simulink model "ddc_dev"  (R2016b)
settings: Solver=VariableStepDiscrete  StartTime=0.0  StopTime=10000  RelTol=1e-3  EnableMultiTasking=on
libraries: xbsIndex_r4 x2641, casper_library_misc x6
(part 6 of 25)

== system ddc_dev/dec_fir1 ==
  sync_in : Inport
  real1 : Inport  Port=2
  imag1 : Inport  Port=3
  real2 : Inport  Port=4
  imag2 : Inport  Port=5
  real3 : Inport  Port=6
  imag3 : Inport  Port=7
  real4 : Inport  Port=8
  imag4 : Inport  Port=9
  real5 : Inport  Port=10
  imag5 : Inport  Port=11
  real6 : Inport  Port=12
  imag6 : Inport  Port=13
  real7 : Inport  Port=14
  imag7 : Inport  Port=15
  real8 : Inport  Port=16
  imag8 : Inport  Port=17
  convert1 : xbsIndex_r4/Convert  gui_display_data_type=Fixed-point  arith_type="Signed  (2's comp)"  n_bits=25  bin_pt=20  float_type=Single  exp_bits=8  fraction_bits=24  quantization="Round  (unbiased: +/- Inf)"  overflow=Wrap  en=off  latency=2  pipeline=off  dbl_ovrd=off  block_type=convert
  convert2 : xbsIndex_r4/Convert  gui_display_data_type=Fixed-point  arith_type="Signed  (2's comp)"  n_bits=25  bin_pt=24  float_type=Single  exp_bits=8  fraction_bits=24  quantization="Round  (unbiased: +/- Inf)"  overflow=Wrap  en=off  latency=2  pipeline=off  dbl_ovrd=off  block_type=convert
  delay : xbsIndex_r4/Delay  rst=off  infoeditControl=Selection of Reset will increase slice count due to use of real FFs and instead of SRLs  en=off  latency=8  reg_retiming=off  dbl_ovrd=off  block_type=delay
      settings: infoedit=Hardware notes: A delay line is a chain, each link of which is an SRL16 or SRL32 followed by a flip-flop.
  fir_dbl_col1 : Subsystem  AncestorBlock=casper_library_downconverter/fir_dbl_col  mask(fir_dbl_col){n_inputs=8, coeff=[-0.0011176 -0.00020448    0.000325  0.00054377  0.00054852  0.00043568  0.00028415  0.00017729], add_latency=1, mult_latency=2, coeff_bit_width=25, coeff_bin_pt=24, first_stage_hdl=on, adder_imp=DSP48}
      mask prompts: n_inputs "Inputs"; coeff "Coefficients"; add_latency "Add latency"; mult_latency "Mult Latency"; coeff_bit_width "Coefficient bit width"; coeff_bin_pt "Coefficient binary point"; first_stage_hdl "Implement first stage of adder trees on output as behavioural HDL"; adder_imp "Adder implementation"
      mask init:
      | fir_dbl_col_init(gcb, ...
      |     'n_inputs', n_inputs, ...
      |     'coeff', coeff, ...
      |     'mult_latency', mult_latency, ...
      |     'add_latency', add_latency, ...
      |     'coeff_bit_width', coeff_bit_width, ...
      |     'coeff_bin_pt', coeff_bin_pt,  ...
      |     'first_stage_hdl', first_stage_hdl, ...
      |     'adder_imp', adder_imp);
      mask Help: eval('xlWeb(''http://casper.berkeley.edu/wiki/Fir_dbl_col'')')
      mask TypeOptions adder_imp: Behavioral | Fabric | DSP48
  fir_dbl_col2 : Subsystem  AncestorBlock=casper_library_downconverter/fir_dbl_col  mask(fir_dbl_col){n_inputs=8, coeff=[-0.0082783  -0.0097532   -0.010008  -0.0092495  -0.0077877  -0.0059668  -0.0041018  -0.0024355], add_latency=1, mult_latency=2, coeff_bit_width=25, coeff_bin_pt=24, first_stage_hdl=on, adder_imp=DSP48}
      mask prompts: n_inputs "Inputs"; coeff "Coefficients"; add_latency "Add latency"; mult_latency "Mult Latency"; coeff_bit_width "Coefficient bit width"; coeff_bin_pt "Coefficient binary point"; first_stage_hdl "Implement first stage of adder trees on output as behavioural HDL"; adder_imp "Adder implementation"
      mask init: same as ddc_dev/dec_fir1/fir_dbl_col1
      mask Help: eval('xlWeb(''http://casper.berkeley.edu/wiki/Fir_dbl_col'')')
      mask TypeOptions adder_imp: Behavioral | Fabric | DSP48
  fir_dbl_col3 : Subsystem  AncestorBlock=casper_library_downconverter/fir_dbl_col  mask(fir_dbl_col){n_inputs=8, coeff=[0.010286    0.012906    0.012956    0.010812   0.0071267   0.0026822  -0.0017544  -0.0055495], add_latency=1, mult_latency=2, coeff_bit_width=25, coeff_bin_pt=24, first_stage_hdl=on, adder_imp=DSP48}
      mask prompts: n_inputs "Inputs"; coeff "Coefficients"; add_latency "Add latency"; mult_latency "Mult Latency"; coeff_bit_width "Coefficient bit width"; coeff_bin_pt "Coefficient binary point"; first_stage_hdl "Implement first stage of adder trees on output as behavioural HDL"; adder_imp "Adder implementation"
      mask init: same as ddc_dev/dec_fir1/fir_dbl_col1
      mask Help: eval('xlWeb(''http://casper.berkeley.edu/wiki/Fir_dbl_col'')')
      mask TypeOptions adder_imp: Behavioral | Fabric | DSP48
  fir_dbl_col4 : Subsystem  AncestorBlock=casper_library_downconverter/fir_dbl_col  mask(fir_dbl_col){n_inputs=8, coeff=[-0.016335   -0.024461   -0.026839   -0.024332   -0.018297   -0.010345  -0.0020805    0.005123], add_latency=1, mult_latency=2, coeff_bit_width=25, coeff_bin_pt=24, first_stage_hdl=on, adder_imp=DSP48}
      mask prompts: n_inputs "Inputs"; coeff "Coefficients"; add_latency "Add latency"; mult_latency "Mult Latency"; coeff_bit_width "Coefficient bit width"; coeff_bin_pt "Coefficient binary point"; first_stage_hdl "Implement first stage of adder trees on output as behavioural HDL"; adder_imp "Adder implementation"
      mask init: same as ddc_dev/dec_fir1/fir_dbl_col1
      mask Help: eval('xlWeb(''http://casper.berkeley.edu/wiki/Fir_dbl_col'')')
      mask TypeOptions adder_imp: Behavioral | Fabric | DSP48
  fir_dbl_col5 : Subsystem  AncestorBlock=casper_library_downconverter/fir_dbl_col  mask(fir_dbl_col){n_inputs=8, coeff=[0.13478      0.1265      0.1109     0.08973    0.065332     0.04028    0.017052  -0.0022894], add_latency=1, mult_latency=2, coeff_bit_width=25, coeff_bin_pt=24, first_stage_hdl=on, adder_imp=DSP48}
      mask prompts: n_inputs "Inputs"; coeff "Coefficients"; add_latency "Add latency"; mult_latency "Mult Latency"; coeff_bit_width "Coefficient bit width"; coeff_bin_pt "Coefficient binary point"; first_stage_hdl "Implement first stage of adder trees on output as behavioural HDL"; adder_imp "Adder implementation"
      mask init: same as ddc_dev/dec_fir1/fir_dbl_col1
      mask Help: eval('xlWeb(''http://casper.berkeley.edu/wiki/Fir_dbl_col'')')
      mask TypeOptions adder_imp: Behavioral | Fabric | DSP48
  imag_sum : Subsystem  AncestorBlock=casper_library_misc/adder_tree  mask(adder_tree){n_inputs=5, latency=1, adder_imp=DSP48, first_stage_hdl=off, floating_point=off, float_type=single, frac_width=0, exp_width=0}
      mask prompts: n_inputs "Number of Inputs"; latency "Add Latency"; adder_imp "Adder implementation"; first_stage_hdl "Use behavioural HDL for first stage of adders"; floating_point "floating point"; float_type "float type"; frac_width "fraction length"; exp_width "exponent length"
      mask help:
      | Sums all inputs using a tree of adds and delays.
      |
      | Number of inputs: The number of inputs to the block to be summed
      | Add latency: The number of clock cycles to perform one addition (affects timing)..
      | Adder implementation: choice of fabric or DSP48E core, or behavioral HDL
      | Use behavioural HDL for first stage of adders: Causes the first stage of adders to be absorbed into DSP blocks if multipliers precede them (Virtex 5). Overrides Adder implementation
      mask init:
      | adder_tree_init(gcb, ...
      |     'n_inputs', n_inputs, ...
      |     'latency', latency, ...
      |     'adder_imp', adder_imp, ...
      |     'floating_point', floating_point, ...
      |     'float_type', float_type, ...
      |     'exp_width', exp_width, ...
      |     'frac_width', frac_width, ...     
      |     'first_stage_hdl', first_stage_hdl);
      settings: AttributesFormatString=latency 3
      mask Help: eval('xlWeb(''http://casper.berkeley.edu/wiki/Adder_tree'')')
      mask TypeOptions adder_imp: Behavioral | Fabric | DSP48
      mask Callback floating_point:
      | onoff = get_param(gcb, 'floating_point');
      | if strcmp(onoff,'on')
      |     enable_fixpt = 'off'
      |     set_param_state(gcb, 'float_type', 'on')
      | 
      |     f_type = get_param(gcb, 'float_type')
      |     if strcmp(f_type,'custom')
      |         set_param_state(gcb, 'exp_width', 'on')
      |         set_param_state(gcb, 'frac_width', 'on')
      |     else
      |         set_param_state(gcb, 'exp_width', 'off')
      |         set_param_state(gcb, 'frac_width', 'off')
      |     end
      | 
      | 
      | else
      |     enable_fixpt = 'on'
      |     set_param_state(gcb, 'float_type', 'off')
      |     set_param_state(gcb, 'exp_width', 'off')
      |     set_param_state(gcb, 'frac_width', 'off')
      | end
      mask TypeOptions float_type: single | custom
      mask Callback float_type:
      | f_type = get_param(gcb, 'float_type')
      | if strcmp(f_type,'custom')
      |     set_param_state(gcb, 'exp_width', 'on')
      |     set_param_state(gcb, 'frac_width', 'on')
      | else
      |     set_param_state(gcb, 'exp_width', 'off')
      |     set_param_state(gcb, 'frac_width', 'off')
      | end
  real_sum : Subsystem  AncestorBlock=casper_library_misc/adder_tree  mask(adder_tree){n_inputs=5, latency=1, adder_imp=DSP48, first_stage_hdl=off, floating_point=off, float_type=single, frac_width=0, exp_width=0}
      mask prompts: n_inputs "Number of Inputs"; latency "Add Latency"; adder_imp "Adder implementation"; first_stage_hdl "Use behavioural HDL for first stage of adders"; floating_point "floating point"; float_type "float type"; frac_width "fraction length"; exp_width "exponent length"
      mask help:
      | Sums all inputs using a tree of adds and delays.
      |
      | Number of inputs: The number of inputs to the block to be summed
      | Add latency: The number of clock cycles to perform one addition (affects timing)..
      | Adder implementation: choice of fabric or DSP48E core, or behavioral HDL
      | Use behavioural HDL for first stage of adders: Causes the first stage of adders to be absorbed into DSP blocks if multipliers precede them (Virtex 5). Overrides Adder implementation
      mask init: same as ddc_dev/dec_fir1/imag_sum
      settings: AttributesFormatString=latency 3
      mask Help: eval('xlWeb(''http://casper.berkeley.edu/wiki/Adder_tree'')')
      mask TypeOptions adder_imp: Behavioral | Fabric | DSP48
      mask Callback floating_point:
      | onoff = get_param(gcb, 'floating_point');
      | if strcmp(onoff,'on')
      |     enable_fixpt = 'off'
      |     set_param_state(gcb, 'float_type', 'on')
      | 
      |     f_type = get_param(gcb, 'float_type')
      |     if strcmp(f_type,'custom')
      |         set_param_state(gcb, 'exp_width', 'on')
      |         set_param_state(gcb, 'frac_width', 'on')
      |     else
      |         set_param_state(gcb, 'exp_width', 'off')
      |         set_param_state(gcb, 'frac_width', 'off')
      |     end
      | 
      | 
      | else
      |     enable_fixpt = 'on'
      |     set_param_state(gcb, 'float_type', 'off')
      |     set_param_state(gcb, 'exp_width', 'off')
      |     set_param_state(gcb, 'frac_width', 'off')
      | end
      mask TypeOptions float_type: single | custom
      mask Callback float_type:
      | f_type = get_param(gcb, 'float_type')
      | if strcmp(f_type,'custom')
      |     set_param_state(gcb, 'exp_width', 'on')
      |     set_param_state(gcb, 'frac_width', 'on')
      | else
      |     set_param_state(gcb, 'exp_width', 'off')
      |     set_param_state(gcb, 'frac_width', 'off')
      | end
  ri_to_c : casper_library_misc/ri_to_c
  shift1 : xbsIndex_r4/Shift  shift_dir=Left  shift_bits=1  en=off  latency=1  precision=Full  arith_type="Signed  (2's comp)"  n_bits=16  bin_pt=14  quantization=Truncate  overflow=Wrap  dbl_ovrd=off  block_type=shift
  shift2 : xbsIndex_r4/Shift  shift_dir=Left  shift_bits=1  en=off  latency=1  precision=Full  arith_type="Signed  (2's comp)"  n_bits=16  bin_pt=14  quantization=Truncate  overflow=Wrap  dbl_ovrd=off  block_type=shift
  sync_out : Outport
  dout : Outport  Port=2
  wires:
  fir_dbl_col5/16(imag_out8) -> fir_dbl_col5/32(imag_back8)
  fir_dbl_col5/15(real_out8) -> fir_dbl_col5/31(real_back8)
  fir_dbl_col5/14(imag_out7) -> fir_dbl_col5/30(imag_back7)
  fir_dbl_col5/13(real_out7) -> fir_dbl_col5/29(real_back7)
  fir_dbl_col5/12(imag_out6) -> fir_dbl_col5/28(imag_back6)
  fir_dbl_col5/11(real_out6) -> fir_dbl_col5/27(real_back6)
  fir_dbl_col5/10(imag_out5) -> fir_dbl_col5/26(imag_back5)
  fir_dbl_col5/9(real_out5) -> fir_dbl_col5/25(real_back5)
  fir_dbl_col5/8(imag_out4) -> fir_dbl_col5/24(imag_back4)
  fir_dbl_col5/7(real_out4) -> fir_dbl_col5/23(real_back4)
  fir_dbl_col5/6(imag_out3) -> fir_dbl_col5/22(imag_back3)
  fir_dbl_col5/5(real_out3) -> fir_dbl_col5/21(real_back3)
  fir_dbl_col5/4(imag_out2) -> fir_dbl_col5/20(imag_back2)
  fir_dbl_col5/3(real_out2) -> fir_dbl_col5/19(real_back2)
  fir_dbl_col5/2(imag_out1) -> fir_dbl_col5/18(imag_back1)
  fir_dbl_col5/1(real_out1) -> fir_dbl_col5/17(real_back1)
  fir_dbl_col5/32(imag_back_out8) -> fir_dbl_col4/32(imag_back8)
  fir_dbl_col5/31(real_back_out8) -> fir_dbl_col4/31(real_back8)
  fir_dbl_col5/30(imag_back_out7) -> fir_dbl_col4/30(imag_back7)
  fir_dbl_col5/29(real_back_out7) -> fir_dbl_col4/29(real_back7)
  fir_dbl_col5/28(imag_back_out6) -> fir_dbl_col4/28(imag_back6)
  fir_dbl_col5/27(real_back_out6) -> fir_dbl_col4/27(real_back6)
  fir_dbl_col5/26(imag_back_out5) -> fir_dbl_col4/26(imag_back5)
  fir_dbl_col5/25(real_back_out5) -> fir_dbl_col4/25(real_back5)
  fir_dbl_col5/24(imag_back_out4) -> fir_dbl_col4/24(imag_back4)
  fir_dbl_col5/23(real_back_out4) -> fir_dbl_col4/23(real_back4)
  fir_dbl_col5/22(imag_back_out3) -> fir_dbl_col4/22(imag_back3)
  fir_dbl_col5/21(real_back_out3) -> fir_dbl_col4/21(real_back3)
  fir_dbl_col5/20(imag_back_out2) -> fir_dbl_col4/20(imag_back2)
  fir_dbl_col5/19(real_back_out2) -> fir_dbl_col4/19(real_back2)
  fir_dbl_col5/18(imag_back_out1) -> fir_dbl_col4/18(imag_back1)
  fir_dbl_col5/17(real_back_out1) -> fir_dbl_col4/17(real_back1)
  fir_dbl_col4/32(imag_back_out8) -> fir_dbl_col3/32(imag_back8)
  fir_dbl_col4/31(real_back_out8) -> fir_dbl_col3/31(real_back8)
  fir_dbl_col4/30(imag_back_out7) -> fir_dbl_col3/30(imag_back7)
  fir_dbl_col4/29(real_back_out7) -> fir_dbl_col3/29(real_back7)
  fir_dbl_col4/28(imag_back_out6) -> fir_dbl_col3/28(imag_back6)
  fir_dbl_col4/27(real_back_out6) -> fir_dbl_col3/27(real_back6)
  fir_dbl_col4/26(imag_back_out5) -> fir_dbl_col3/26(imag_back5)
  fir_dbl_col4/25(real_back_out5) -> fir_dbl_col3/25(real_back5)
  fir_dbl_col4/24(imag_back_out4) -> fir_dbl_col3/24(imag_back4)
  fir_dbl_col4/23(real_back_out4) -> fir_dbl_col3/23(real_back4)
  fir_dbl_col4/22(imag_back_out3) -> fir_dbl_col3/22(imag_back3)
  fir_dbl_col4/21(real_back_out3) -> fir_dbl_col3/21(real_back3)
  fir_dbl_col4/20(imag_back_out2) -> fir_dbl_col3/20(imag_back2)
  fir_dbl_col4/19(real_back_out2) -> fir_dbl_col3/19(real_back2)
  fir_dbl_col4/18(imag_back_out1) -> fir_dbl_col3/18(imag_back1)
  fir_dbl_col4/17(real_back_out1) -> fir_dbl_col3/17(real_back1)
  fir_dbl_col3/32(imag_back_out8) -> fir_dbl_col2/32(imag_back8)
  fir_dbl_col3/31(real_back_out8) -> fir_dbl_col2/31(real_back8)
  fir_dbl_col3/30(imag_back_out7) -> fir_dbl_col2/30(imag_back7)
  fir_dbl_col3/29(real_back_out7) -> fir_dbl_col2/29(real_back7)
  fir_dbl_col3/28(imag_back_out6) -> fir_dbl_col2/28(imag_back6)
  fir_dbl_col3/27(real_back_out6) -> fir_dbl_col2/27(real_back6)
  fir_dbl_col3/26(imag_back_out5) -> fir_dbl_col2/26(imag_back5)
  fir_dbl_col3/25(real_back_out5) -> fir_dbl_col2/25(real_back5)
  fir_dbl_col3/24(imag_back_out4) -> fir_dbl_col2/24(imag_back4)
  fir_dbl_col3/23(real_back_out4) -> fir_dbl_col2/23(real_back4)
  fir_dbl_col3/22(imag_back_out3) -> fir_dbl_col2/22(imag_back3)
  fir_dbl_col3/21(real_back_out3) -> fir_dbl_col2/21(real_back3)
  fir_dbl_col3/20(imag_back_out2) -> fir_dbl_col2/20(imag_back2)
  fir_dbl_col3/19(real_back_out2) -> fir_dbl_col2/19(real_back2)
  fir_dbl_col3/18(imag_back_out1) -> fir_dbl_col2/18(imag_back1)
  fir_dbl_col3/17(real_back_out1) -> fir_dbl_col2/17(real_back1)
  fir_dbl_col2/32(imag_back_out8) -> fir_dbl_col1/32(imag_back8)
  fir_dbl_col2/31(real_back_out8) -> fir_dbl_col1/31(real_back8)
  fir_dbl_col2/30(imag_back_out7) -> fir_dbl_col1/30(imag_back7)
  fir_dbl_col2/29(real_back_out7) -> fir_dbl_col1/29(real_back7)
  fir_dbl_col2/28(imag_back_out6) -> fir_dbl_col1/28(imag_back6)
  fir_dbl_col2/27(real_back_out6) -> fir_dbl_col1/27(real_back6)
  fir_dbl_col2/26(imag_back_out5) -> fir_dbl_col1/26(imag_back5)
  fir_dbl_col2/25(real_back_out5) -> fir_dbl_col1/25(real_back5)
  fir_dbl_col2/24(imag_back_out4) -> fir_dbl_col1/24(imag_back4)
  fir_dbl_col2/23(real_back_out4) -> fir_dbl_col1/23(real_back4)
  fir_dbl_col2/22(imag_back_out3) -> fir_dbl_col1/22(imag_back3)
  fir_dbl_col2/21(real_back_out3) -> fir_dbl_col1/21(real_back3)
  fir_dbl_col2/20(imag_back_out2) -> fir_dbl_col1/20(imag_back2)
  fir_dbl_col2/19(real_back_out2) -> fir_dbl_col1/19(real_back2)
  fir_dbl_col2/18(imag_back_out1) -> fir_dbl_col1/18(imag_back1)
  fir_dbl_col2/17(real_back_out1) -> fir_dbl_col1/17(real_back1)
  real_sum/1(sync_out) -> sync_out/1
  delay/1 -> imag_sum/1(sync), real_sum/1(sync)
  sync_in/1 -> delay/1
  ri_to_c/1 -> dout/1
  convert2/1 -> ri_to_c/2
  convert1/1 -> ri_to_c/1
  shift2/1 -> convert2/1
  shift1/1 -> convert1/1
  imag_sum/2(dout) -> shift2/1
  real_sum/2(dout) -> shift1/1
  fir_dbl_col5/34(imag_sum) -> imag_sum/6(din5)
  fir_dbl_col5/33(real_sum) -> real_sum/6(din5)
  fir_dbl_col4/16(imag_out8) -> fir_dbl_col5/16(imag8)
  fir_dbl_col4/15(real_out8) -> fir_dbl_col5/15(real8)
  fir_dbl_col4/14(imag_out7) -> fir_dbl_col5/14(imag7)
  fir_dbl_col4/13(real_out7) -> fir_dbl_col5/13(real7)
  fir_dbl_col4/12(imag_out6) -> fir_dbl_col5/12(imag6)
  fir_dbl_col4/11(real_out6) -> fir_dbl_col5/11(real6)
  fir_dbl_col4/10(imag_out5) -> fir_dbl_col5/10(imag5)
  fir_dbl_col4/9(real_out5) -> fir_dbl_col5/9(real5)
  fir_dbl_col4/8(imag_out4) -> fir_dbl_col5/8(imag4)
  fir_dbl_col4/7(real_out4) -> fir_dbl_col5/7(real4)
  fir_dbl_col4/6(imag_out3) -> fir_dbl_col5/6(imag3)
  fir_dbl_col4/5(real_out3) -> fir_dbl_col5/5(real3)
  fir_dbl_col4/4(imag_out2) -> fir_dbl_col5/4(imag2)
  fir_dbl_col4/3(real_out2) -> fir_dbl_col5/3(real2)
  fir_dbl_col4/2(imag_out1) -> fir_dbl_col5/2(imag1)
  fir_dbl_col4/1(real_out1) -> fir_dbl_col5/1(real1)
  fir_dbl_col4/34(imag_sum) -> imag_sum/5(din4)
  fir_dbl_col4/33(real_sum) -> real_sum/5(din4)
  fir_dbl_col3/16(imag_out8) -> fir_dbl_col4/16(imag8)
  fir_dbl_col3/15(real_out8) -> fir_dbl_col4/15(real8)
  fir_dbl_col3/14(imag_out7) -> fir_dbl_col4/14(imag7)
  fir_dbl_col3/13(real_out7) -> fir_dbl_col4/13(real7)
  fir_dbl_col3/12(imag_out6) -> fir_dbl_col4/12(imag6)
  fir_dbl_col3/11(real_out6) -> fir_dbl_col4/11(real6)
  fir_dbl_col3/10(imag_out5) -> fir_dbl_col4/10(imag5)
  fir_dbl_col3/9(real_out5) -> fir_dbl_col4/9(real5)
  fir_dbl_col3/8(imag_out4) -> fir_dbl_col4/8(imag4)
  fir_dbl_col3/7(real_out4) -> fir_dbl_col4/7(real4)
  fir_dbl_col3/6(imag_out3) -> fir_dbl_col4/6(imag3)
  fir_dbl_col3/5(real_out3) -> fir_dbl_col4/5(real3)
  fir_dbl_col3/4(imag_out2) -> fir_dbl_col4/4(imag2)
  fir_dbl_col3/3(real_out2) -> fir_dbl_col4/3(real2)
  fir_dbl_col3/2(imag_out1) -> fir_dbl_col4/2(imag1)
  fir_dbl_col3/1(real_out1) -> fir_dbl_col4/1(real1)
  fir_dbl_col3/34(imag_sum) -> imag_sum/4(din3)
  fir_dbl_col3/33(real_sum) -> real_sum/4(din3)
  fir_dbl_col2/16(imag_out8) -> fir_dbl_col3/16(imag8)
  fir_dbl_col2/15(real_out8) -> fir_dbl_col3/15(real8)
  fir_dbl_col2/14(imag_out7) -> fir_dbl_col3/14(imag7)
  fir_dbl_col2/13(real_out7) -> fir_dbl_col3/13(real7)
  fir_dbl_col2/12(imag_out6) -> fir_dbl_col3/12(imag6)
  fir_dbl_col2/11(real_out6) -> fir_dbl_col3/11(real6)
  fir_dbl_col2/10(imag_out5) -> fir_dbl_col3/10(imag5)
  fir_dbl_col2/9(real_out5) -> fir_dbl_col3/9(real5)
  fir_dbl_col2/8(imag_out4) -> fir_dbl_col3/8(imag4)
  fir_dbl_col2/7(real_out4) -> fir_dbl_col3/7(real4)
  fir_dbl_col2/6(imag_out3) -> fir_dbl_col3/6(imag3)
  fir_dbl_col2/5(real_out3) -> fir_dbl_col3/5(real3)
  fir_dbl_col2/4(imag_out2) -> fir_dbl_col3/4(imag2)
  fir_dbl_col2/3(real_out2) -> fir_dbl_col3/3(real2)
  fir_dbl_col2/2(imag_out1) -> fir_dbl_col3/2(imag1)
  fir_dbl_col2/1(real_out1) -> fir_dbl_col3/1(real1)
  fir_dbl_col2/34(imag_sum) -> imag_sum/3(din2)
  fir_dbl_col2/33(real_sum) -> real_sum/3(din2)
  fir_dbl_col1/16(imag_out8) -> fir_dbl_col2/16(imag8)
  fir_dbl_col1/15(real_out8) -> fir_dbl_col2/15(real8)
  fir_dbl_col1/14(imag_out7) -> fir_dbl_col2/14(imag7)
  fir_dbl_col1/13(real_out7) -> fir_dbl_col2/13(real7)
  fir_dbl_col1/12(imag_out6) -> fir_dbl_col2/12(imag6)
  fir_dbl_col1/11(real_out6) -> fir_dbl_col2/11(real6)
  fir_dbl_col1/10(imag_out5) -> fir_dbl_col2/10(imag5)
  fir_dbl_col1/9(real_out5) -> fir_dbl_col2/9(real5)
  fir_dbl_col1/8(imag_out4) -> fir_dbl_col2/8(imag4)
  fir_dbl_col1/7(real_out4) -> fir_dbl_col2/7(real4)
  fir_dbl_col1/6(imag_out3) -> fir_dbl_col2/6(imag3)
  fir_dbl_col1/5(real_out3) -> fir_dbl_col2/5(real3)
  fir_dbl_col1/4(imag_out2) -> fir_dbl_col2/4(imag2)
  fir_dbl_col1/3(real_out2) -> fir_dbl_col2/3(real2)
  fir_dbl_col1/2(imag_out1) -> fir_dbl_col2/2(imag1)
  fir_dbl_col1/1(real_out1) -> fir_dbl_col2/1(real1)
  fir_dbl_col1/34(imag_sum) -> imag_sum/2(din1)
  fir_dbl_col1/33(real_sum) -> real_sum/2(din1)
  imag8/1 -> fir_dbl_col1/16(imag8)
  real8/1 -> fir_dbl_col1/15(real8)
  imag7/1 -> fir_dbl_col1/14(imag7)
  real7/1 -> fir_dbl_col1/13(real7)
  imag6/1 -> fir_dbl_col1/12(imag6)
  real6/1 -> fir_dbl_col1/11(real6)
  imag5/1 -> fir_dbl_col1/10(imag5)
  real5/1 -> fir_dbl_col1/9(real5)
  imag4/1 -> fir_dbl_col1/8(imag4)
  real4/1 -> fir_dbl_col1/7(real4)
  imag3/1 -> fir_dbl_col1/6(imag3)
  real3/1 -> fir_dbl_col1/5(real3)
  imag2/1 -> fir_dbl_col1/4(imag2)
  real2/1 -> fir_dbl_col1/3(real2)
  imag1/1 -> fir_dbl_col1/2(imag1)
  real1/1 -> fir_dbl_col1/1(real1)

== system ddc_dev/dec_fir2 ==
  sync_in : Inport
  real1 : Inport  Port=2
  imag1 : Inport  Port=3
  real2 : Inport  Port=4
  imag2 : Inport  Port=5
  real3 : Inport  Port=6
  imag3 : Inport  Port=7
  real4 : Inport  Port=8
  imag4 : Inport  Port=9
  real5 : Inport  Port=10
  imag5 : Inport  Port=11
  real6 : Inport  Port=12
  imag6 : Inport  Port=13
  real7 : Inport  Port=14
  imag7 : Inport  Port=15
  real8 : Inport  Port=16
  imag8 : Inport  Port=17
  convert1 : xbsIndex_r4/Convert  gui_display_data_type=Fixed-point  arith_type="Signed  (2's comp)"  n_bits=25  bin_pt=20  float_type=Single  exp_bits=8  fraction_bits=24  quantization="Round  (unbiased: +/- Inf)"  overflow=Wrap  en=off  latency=2  pipeline=off  dbl_ovrd=off  block_type=convert
  convert2 : xbsIndex_r4/Convert  gui_display_data_type=Fixed-point  arith_type="Signed  (2's comp)"  n_bits=25  bin_pt=24  float_type=Single  exp_bits=8  fraction_bits=24  quantization="Round  (unbiased: +/- Inf)"  overflow=Wrap  en=off  latency=2  pipeline=off  dbl_ovrd=off  block_type=convert
  delay : xbsIndex_r4/Delay  rst=off  infoeditControl=Selection of Reset will increase slice count due to use of real FFs and instead of SRLs  en=off  latency=8  reg_retiming=off  dbl_ovrd=off  block_type=delay
      settings: infoedit=Hardware notes: A delay line is a chain, each link of which is an SRL16 or SRL32 followed by a flip-flop.
  fir_dbl_col1 : Subsystem  AncestorBlock=casper_library_downconverter/fir_dbl_col  mask(fir_dbl_col){n_inputs=8, coeff=[-0.0011176 -0.00020448    0.000325  0.00054377  0.00054852  0.00043568  0.00028415  0.00017729], add_latency=1, mult_latency=2, coeff_bit_width=25, coeff_bin_pt=24, first_stage_hdl=on, adder_imp=DSP48}
      mask prompts: n_inputs "Inputs"; coeff "Coefficients"; add_latency "Add latency"; mult_latency "Mult Latency"; coeff_bit_width "Coefficient bit width"; coeff_bin_pt "Coefficient binary point"; first_stage_hdl "Implement first stage of adder trees on output as behavioural HDL"; adder_imp "Adder implementation"
      mask init: same as ddc_dev/dec_fir1/fir_dbl_col1
      mask Help: eval('xlWeb(''http://casper.berkeley.edu/wiki/Fir_dbl_col'')')
      mask TypeOptions adder_imp: Behavioral | Fabric | DSP48
  fir_dbl_col2 : Subsystem  AncestorBlock=casper_library_downconverter/fir_dbl_col  mask(fir_dbl_col){n_inputs=8, coeff=[-0.0082783  -0.0097532   -0.010008  -0.0092495  -0.0077877  -0.0059668  -0.0041018  -0.0024355], add_latency=1, mult_latency=2, coeff_bit_width=25, coeff_bin_pt=24, first_stage_hdl=on, adder_imp=DSP48}
      mask prompts: n_inputs "Inputs"; coeff "Coefficients"; add_latency "Add latency"; mult_latency "Mult Latency"; coeff_bit_width "Coefficient bit width"; coeff_bin_pt "Coefficient binary point"; first_stage_hdl "Implement first stage of adder trees on output as behavioural HDL"; adder_imp "Adder implementation"
      mask init: same as ddc_dev/dec_fir1/fir_dbl_col1
      mask Help: eval('xlWeb(''http://casper.berkeley.edu/wiki/Fir_dbl_col'')')
      mask TypeOptions adder_imp: Behavioral | Fabric | DSP48
  fir_dbl_col3 : Subsystem  AncestorBlock=casper_library_downconverter/fir_dbl_col  mask(fir_dbl_col){n_inputs=8, coeff=[0.010286    0.012906    0.012956    0.010812   0.0071267   0.0026822  -0.0017544  -0.0055495], add_latency=1, mult_latency=2, coeff_bit_width=25, coeff_bin_pt=24, first_stage_hdl=on, adder_imp=DSP48}
      mask prompts: n_inputs "Inputs"; coeff "Coefficients"; add_latency "Add latency"; mult_latency "Mult Latency"; coeff_bit_width "Coefficient bit width"; coeff_bin_pt "Coefficient binary point"; first_stage_hdl "Implement first stage of adder trees on output as behavioural HDL"; adder_imp "Adder implementation"
      mask init: same as ddc_dev/dec_fir1/fir_dbl_col1
      mask Help: eval('xlWeb(''http://casper.berkeley.edu/wiki/Fir_dbl_col'')')
      mask TypeOptions adder_imp: Behavioral | Fabric | DSP48
  fir_dbl_col4 : Subsystem  AncestorBlock=casper_library_downconverter/fir_dbl_col  mask(fir_dbl_col){n_inputs=8, coeff=[-0.016335   -0.024461   -0.026839   -0.024332   -0.018297   -0.010345  -0.0020805    0.005123], add_latency=1, mult_latency=2, coeff_bit_width=25, coeff_bin_pt=24, first_stage_hdl=on, adder_imp=DSP48}
      mask prompts: n_inputs "Inputs"; coeff "Coefficients"; add_latency "Add latency"; mult_latency "Mult Latency"; coeff_bit_width "Coefficient bit width"; coeff_bin_pt "Coefficient binary point"; first_stage_hdl "Implement first stage of adder trees on output as behavioural HDL"; adder_imp "Adder implementation"
      mask init: same as ddc_dev/dec_fir1/fir_dbl_col1
      mask Help: eval('xlWeb(''http://casper.berkeley.edu/wiki/Fir_dbl_col'')')
      mask TypeOptions adder_imp: Behavioral | Fabric | DSP48
  fir_dbl_col5 : Subsystem  AncestorBlock=casper_library_downconverter/fir_dbl_col  mask(fir_dbl_col){n_inputs=8, coeff=[0.13478      0.1265      0.1109     0.08973    0.065332     0.04028    0.017052  -0.0022894], add_latency=1, mult_latency=2, coeff_bit_width=25, coeff_bin_pt=24, first_stage_hdl=on, adder_imp=DSP48}
      mask prompts: n_inputs "Inputs"; coeff "Coefficients"; add_latency "Add latency"; mult_latency "Mult Latency"; coeff_bit_width "Coefficient bit width"; coeff_bin_pt "Coefficient binary point"; first_stage_hdl "Implement first stage of adder trees on output as behavioural HDL"; adder_imp "Adder implementation"
      mask init: same as ddc_dev/dec_fir1/fir_dbl_col1
      mask Help: eval('xlWeb(''http://casper.berkeley.edu/wiki/Fir_dbl_col'')')
      mask TypeOptions adder_imp: Behavioral | Fabric | DSP48
  imag_sum : Subsystem  AncestorBlock=casper_library_misc/adder_tree  mask(adder_tree){n_inputs=5, latency=1, adder_imp=DSP48, first_stage_hdl=off, floating_point=off, float_type=single, frac_width=0, exp_width=0}
      mask prompts: n_inputs "Number of Inputs"; latency "Add Latency"; adder_imp "Adder implementation"; first_stage_hdl "Use behavioural HDL for first stage of adders"; floating_point "floating point"; float_type "float type"; frac_width "fraction length"; exp_width "exponent length"
      mask help:
      | Sums all inputs using a tree of adds and delays.
      |
      | Number of inputs: The number of inputs to the block to be summed
      | Add latency: The number of clock cycles to perform one addition (affects timing)..
      | Adder implementation: choice of fabric or DSP48E core, or behavioral HDL
      | Use behavioural HDL for first stage of adders: Causes the first stage of adders to be absorbed into DSP blocks if multipliers precede them (Virtex 5). Overrides Adder implementation
      mask init: same as ddc_dev/dec_fir1/imag_sum
      settings: AttributesFormatString=latency 3
      mask Help: eval('xlWeb(''http://casper.berkeley.edu/wiki/Adder_tree'')')
      mask TypeOptions adder_imp: Behavioral | Fabric | DSP48
      mask Callback floating_point:
      | onoff = get_param(gcb, 'floating_point');
      | if strcmp(onoff,'on')
      |     enable_fixpt = 'off'
      |     set_param_state(gcb, 'float_type', 'on')
      | 
      |     f_type = get_param(gcb, 'float_type')
      |     if strcmp(f_type,'custom')
      |         set_param_state(gcb, 'exp_width', 'on')
      |         set_param_state(gcb, 'frac_width', 'on')
      |     else
      |         set_param_state(gcb, 'exp_width', 'off')
      |         set_param_state(gcb, 'frac_width', 'off')
      |     end
      | 
      | 
      | else
      |     enable_fixpt = 'on'
      |     set_param_state(gcb, 'float_type', 'off')
      |     set_param_state(gcb, 'exp_width', 'off')
      |     set_param_state(gcb, 'frac_width', 'off')
      | end
      mask TypeOptions float_type: single | custom
      mask Callback float_type:
      | f_type = get_param(gcb, 'float_type')
      | if strcmp(f_type,'custom')
      |     set_param_state(gcb, 'exp_width', 'on')
      |     set_param_state(gcb, 'frac_width', 'on')
      | else
      |     set_param_state(gcb, 'exp_width', 'off')
      |     set_param_state(gcb, 'frac_width', 'off')
      | end
  real_sum : Subsystem  AncestorBlock=casper_library_misc/adder_tree  mask(adder_tree){n_inputs=5, latency=1, adder_imp=DSP48, first_stage_hdl=off, floating_point=off, float_type=single, frac_width=0, exp_width=0}
      mask prompts: n_inputs "Number of Inputs"; latency "Add Latency"; adder_imp "Adder implementation"; first_stage_hdl "Use behavioural HDL for first stage of adders"; floating_point "floating point"; float_type "float type"; frac_width "fraction length"; exp_width "exponent length"
      mask help:
      | Sums all inputs using a tree of adds and delays.
      |
      | Number of inputs: The number of inputs to the block to be summed
      | Add latency: The number of clock cycles to perform one addition (affects timing)..
      | Adder implementation: choice of fabric or DSP48E core, or behavioral HDL
      | Use behavioural HDL for first stage of adders: Causes the first stage of adders to be absorbed into DSP blocks if multipliers precede them (Virtex 5). Overrides Adder implementation
      mask init: same as ddc_dev/dec_fir1/imag_sum
      settings: AttributesFormatString=latency 3
      mask Help: eval('xlWeb(''http://casper.berkeley.edu/wiki/Adder_tree'')')
      mask TypeOptions adder_imp: Behavioral | Fabric | DSP48
      mask Callback floating_point:
      | onoff = get_param(gcb, 'floating_point');
      | if strcmp(onoff,'on')
      |     enable_fixpt = 'off'
      |     set_param_state(gcb, 'float_type', 'on')
      | 
      |     f_type = get_param(gcb, 'float_type')
      |     if strcmp(f_type,'custom')
      |         set_param_state(gcb, 'exp_width', 'on')
      |         set_param_state(gcb, 'frac_width', 'on')
      |     else
      |         set_param_state(gcb, 'exp_width', 'off')
      |         set_param_state(gcb, 'frac_width', 'off')
      |     end
      | 
      | 
      | else
      |     enable_fixpt = 'on'
      |     set_param_state(gcb, 'float_type', 'off')
      |     set_param_state(gcb, 'exp_width', 'off')
      |     set_param_state(gcb, 'frac_width', 'off')
      | end
      mask TypeOptions float_type: single | custom
      mask Callback float_type:
      | f_type = get_param(gcb, 'float_type')
      | if strcmp(f_type,'custom')
      |     set_param_state(gcb, 'exp_width', 'on')
      |     set_param_state(gcb, 'frac_width', 'on')
      | else
      |     set_param_state(gcb, 'exp_width', 'off')
      |     set_param_state(gcb, 'frac_width', 'off')
      | end
  ri_to_c : casper_library_misc/ri_to_c
  shift1 : xbsIndex_r4/Shift  shift_dir=Left  shift_bits=1  en=off  latency=1  precision=Full  arith_type="Signed  (2's comp)"  n_bits=16  bin_pt=14  quantization=Truncate  overflow=Wrap  dbl_ovrd=off  block_type=shift
  shift2 : xbsIndex_r4/Shift  shift_dir=Left  shift_bits=1  en=off  latency=1  precision=Full  arith_type="Signed  (2's comp)"  n_bits=16  bin_pt=14  quantization=Truncate  overflow=Wrap  dbl_ovrd=off  block_type=shift
  sync_out : Outport
  dout : Outport  Port=2
  wires:
  real1/1 -> fir_dbl_col1/1(real1)
  imag1/1 -> fir_dbl_col1/2(imag1)
  real2/1 -> fir_dbl_col1/3(real2)
  imag2/1 -> fir_dbl_col1/4(imag2)
  real3/1 -> fir_dbl_col1/5(real3)
  imag3/1 -> fir_dbl_col1/6(imag3)
  real4/1 -> fir_dbl_col1/7(real4)
  imag4/1 -> fir_dbl_col1/8(imag4)
  real5/1 -> fir_dbl_col1/9(real5)
  imag5/1 -> fir_dbl_col1/10(imag5)
  real6/1 -> fir_dbl_col1/11(real6)
  imag6/1 -> fir_dbl_col1/12(imag6)
  real7/1 -> fir_dbl_col1/13(real7)
  imag7/1 -> fir_dbl_col1/14(imag7)
  real8/1 -> fir_dbl_col1/15(real8)
  imag8/1 -> fir_dbl_col1/16(imag8)
  fir_dbl_col1/33(real_sum) -> real_sum/2(din1)
  fir_dbl_col1/34(imag_sum) -> imag_sum/2(din1)
  fir_dbl_col1/1(real_out1) -> fir_dbl_col2/1(real1)
  fir_dbl_col1/2(imag_out1) -> fir_dbl_col2/2(imag1)
  fir_dbl_col1/3(real_out2) -> fir_dbl_col2/3(real2)
  fir_dbl_col1/4(imag_out2) -> fir_dbl_col2/4(imag2)
  fir_dbl_col1/5(real_out3) -> fir_dbl_col2/5(real3)
  fir_dbl_col1/6(imag_out3) -> fir_dbl_col2/6(imag3)
  fir_dbl_col1/7(real_out4) -> fir_dbl_col2/7(real4)
  fir_dbl_col1/8(imag_out4) -> fir_dbl_col2/8(imag4)
  fir_dbl_col1/9(real_out5) -> fir_dbl_col2/9(real5)
  fir_dbl_col1/10(imag_out5) -> fir_dbl_col2/10(imag5)
  fir_dbl_col1/11(real_out6) -> fir_dbl_col2/11(real6)
  fir_dbl_col1/12(imag_out6) -> fir_dbl_col2/12(imag6)
  fir_dbl_col1/13(real_out7) -> fir_dbl_col2/13(real7)
  fir_dbl_col1/14(imag_out7) -> fir_dbl_col2/14(imag7)
  fir_dbl_col1/15(real_out8) -> fir_dbl_col2/15(real8)
  fir_dbl_col1/16(imag_out8) -> fir_dbl_col2/16(imag8)
  fir_dbl_col2/33(real_sum) -> real_sum/3(din2)
  fir_dbl_col2/34(imag_sum) -> imag_sum/3(din2)
  fir_dbl_col2/1(real_out1) -> fir_dbl_col3/1(real1)
  fir_dbl_col2/2(imag_out1) -> fir_dbl_col3/2(imag1)
  fir_dbl_col2/3(real_out2) -> fir_dbl_col3/3(real2)
  fir_dbl_col2/4(imag_out2) -> fir_dbl_col3/4(imag2)
  fir_dbl_col2/5(real_out3) -> fir_dbl_col3/5(real3)
  fir_dbl_col2/6(imag_out3) -> fir_dbl_col3/6(imag3)
  fir_dbl_col2/7(real_out4) -> fir_dbl_col3/7(real4)
  fir_dbl_col2/8(imag_out4) -> fir_dbl_col3/8(imag4)
  fir_dbl_col2/9(real_out5) -> fir_dbl_col3/9(real5)
  fir_dbl_col2/10(imag_out5) -> fir_dbl_col3/10(imag5)
  fir_dbl_col2/11(real_out6) -> fir_dbl_col3/11(real6)
  fir_dbl_col2/12(imag_out6) -> fir_dbl_col3/12(imag6)
  fir_dbl_col2/13(real_out7) -> fir_dbl_col3/13(real7)
  fir_dbl_col2/14(imag_out7) -> fir_dbl_col3/14(imag7)
  fir_dbl_col2/15(real_out8) -> fir_dbl_col3/15(real8)
  fir_dbl_col2/16(imag_out8) -> fir_dbl_col3/16(imag8)
  fir_dbl_col3/33(real_sum) -> real_sum/4(din3)
  fir_dbl_col3/34(imag_sum) -> imag_sum/4(din3)
  fir_dbl_col3/1(real_out1) -> fir_dbl_col4/1(real1)
  fir_dbl_col3/2(imag_out1) -> fir_dbl_col4/2(imag1)
  fir_dbl_col3/3(real_out2) -> fir_dbl_col4/3(real2)
  fir_dbl_col3/4(imag_out2) -> fir_dbl_col4/4(imag2)
  fir_dbl_col3/5(real_out3) -> fir_dbl_col4/5(real3)
  fir_dbl_col3/6(imag_out3) -> fir_dbl_col4/6(imag3)
  fir_dbl_col3/7(real_out4) -> fir_dbl_col4/7(real4)
  fir_dbl_col3/8(imag_out4) -> fir_dbl_col4/8(imag4)
  fir_dbl_col3/9(real_out5) -> fir_dbl_col4/9(real5)
  fir_dbl_col3/10(imag_out5) -> fir_dbl_col4/10(imag5)
  fir_dbl_col3/11(real_out6) -> fir_dbl_col4/11(real6)
  fir_dbl_col3/12(imag_out6) -> fir_dbl_col4/12(imag6)
  fir_dbl_col3/13(real_out7) -> fir_dbl_col4/13(real7)
  fir_dbl_col3/14(imag_out7) -> fir_dbl_col4/14(imag7)
  fir_dbl_col3/15(real_out8) -> fir_dbl_col4/15(real8)
  fir_dbl_col3/16(imag_out8) -> fir_dbl_col4/16(imag8)
  fir_dbl_col4/33(real_sum) -> real_sum/5(din4)
  fir_dbl_col4/34(imag_sum) -> imag_sum/5(din4)
  fir_dbl_col4/1(real_out1) -> fir_dbl_col5/1(real1)
  fir_dbl_col4/2(imag_out1) -> fir_dbl_col5/2(imag1)
  fir_dbl_col4/3(real_out2) -> fir_dbl_col5/3(real2)
  fir_dbl_col4/4(imag_out2) -> fir_dbl_col5/4(imag2)
  fir_dbl_col4/5(real_out3) -> fir_dbl_col5/5(real3)
  fir_dbl_col4/6(imag_out3) -> fir_dbl_col5/6(imag3)
  fir_dbl_col4/7(real_out4) -> fir_dbl_col5/7(real4)
  fir_dbl_col4/8(imag_out4) -> fir_dbl_col5/8(imag4)
  fir_dbl_col4/9(real_out5) -> fir_dbl_col5/9(real5)
  fir_dbl_col4/10(imag_out5) -> fir_dbl_col5/10(imag5)
  fir_dbl_col4/11(real_out6) -> fir_dbl_col5/11(real6)
  fir_dbl_col4/12(imag_out6) -> fir_dbl_col5/12(imag6)
  fir_dbl_col4/13(real_out7) -> fir_dbl_col5/13(real7)
  fir_dbl_col4/14(imag_out7) -> fir_dbl_col5/14(imag7)
  fir_dbl_col4/15(real_out8) -> fir_dbl_col5/15(real8)
  fir_dbl_col4/16(imag_out8) -> fir_dbl_col5/16(imag8)
  fir_dbl_col5/33(real_sum) -> real_sum/6(din5)
  fir_dbl_col5/34(imag_sum) -> imag_sum/6(din5)
  real_sum/2(dout) -> shift1/1
  imag_sum/2(dout) -> shift2/1
  shift1/1 -> convert1/1
  shift2/1 -> convert2/1
  convert1/1 -> ri_to_c/1
  convert2/1 -> ri_to_c/2
  ri_to_c/1 -> dout/1
  sync_in/1 -> delay/1
  delay/1 -> real_sum/1(sync), imag_sum/1(sync)
  real_sum/1(sync_out) -> sync_out/1
  fir_dbl_col2/17(real_back_out1) -> fir_dbl_col1/17(real_back1)
  fir_dbl_col2/18(imag_back_out1) -> fir_dbl_col1/18(imag_back1)
  fir_dbl_col2/19(real_back_out2) -> fir_dbl_col1/19(real_back2)
  fir_dbl_col2/20(imag_back_out2) -> fir_dbl_col1/20(imag_back2)
  fir_dbl_col2/21(real_back_out3) -> fir_dbl_col1/21(real_back3)
  fir_dbl_col2/22(imag_back_out3) -> fir_dbl_col1/22(imag_back3)
  fir_dbl_col2/23(real_back_out4) -> fir_dbl_col1/23(real_back4)
  fir_dbl_col2/24(imag_back_out4) -> fir_dbl_col1/24(imag_back4)
  fir_dbl_col2/25(real_back_out5) -> fir_dbl_col1/25(real_back5)
  fir_dbl_col2/26(imag_back_out5) -> fir_dbl_col1/26(imag_back5)
  fir_dbl_col2/27(real_back_out6) -> fir_dbl_col1/27(real_back6)
  fir_dbl_col2/28(imag_back_out6) -> fir_dbl_col1/28(imag_back6)
  fir_dbl_col2/29(real_back_out7) -> fir_dbl_col1/29(real_back7)
  fir_dbl_col2/30(imag_back_out7) -> fir_dbl_col1/30(imag_back7)
  fir_dbl_col2/31(real_back_out8) -> fir_dbl_col1/31(real_back8)
  fir_dbl_col2/32(imag_back_out8) -> fir_dbl_col1/32(imag_back8)
  fir_dbl_col3/17(real_back_out1) -> fir_dbl_col2/17(real_back1)
  fir_dbl_col3/18(imag_back_out1) -> fir_dbl_col2/18(imag_back1)
  fir_dbl_col3/19(real_back_out2) -> fir_dbl_col2/19(real_back2)
  fir_dbl_col3/20(imag_back_out2) -> fir_dbl_col2/20(imag_back2)
  fir_dbl_col3/21(real_back_out3) -> fir_dbl_col2/21(real_back3)
  fir_dbl_col3/22(imag_back_out3) -> fir_dbl_col2/22(imag_back3)
  fir_dbl_col3/23(real_back_out4) -> fir_dbl_col2/23(real_back4)
  fir_dbl_col3/24(imag_back_out4) -> fir_dbl_col2/24(imag_back4)
  fir_dbl_col3/25(real_back_out5) -> fir_dbl_col2/25(real_back5)
  fir_dbl_col3/26(imag_back_out5) -> fir_dbl_col2/26(imag_back5)
  fir_dbl_col3/27(real_back_out6) -> fir_dbl_col2/27(real_back6)
  fir_dbl_col3/28(imag_back_out6) -> fir_dbl_col2/28(imag_back6)
  fir_dbl_col3/29(real_back_out7) -> fir_dbl_col2/29(real_back7)
  fir_dbl_col3/30(imag_back_out7) -> fir_dbl_col2/30(imag_back7)
  fir_dbl_col3/31(real_back_out8) -> fir_dbl_col2/31(real_back8)
  fir_dbl_col3/32(imag_back_out8) -> fir_dbl_col2/32(imag_back8)
  fir_dbl_col4/17(real_back_out1) -> fir_dbl_col3/17(real_back1)
  fir_dbl_col4/18(imag_back_out1) -> fir_dbl_col3/18(imag_back1)
  fir_dbl_col4/19(real_back_out2) -> fir_dbl_col3/19(real_back2)
  fir_dbl_col4/20(imag_back_out2) -> fir_dbl_col3/20(imag_back2)
  fir_dbl_col4/21(real_back_out3) -> fir_dbl_col3/21(real_back3)
  fir_dbl_col4/22(imag_back_out3) -> fir_dbl_col3/22(imag_back3)
  fir_dbl_col4/23(real_back_out4) -> fir_dbl_col3/23(real_back4)
  fir_dbl_col4/24(imag_back_out4) -> fir_dbl_col3/24(imag_back4)
  fir_dbl_col4/25(real_back_out5) -> fir_dbl_col3/25(real_back5)
  fir_dbl_col4/26(imag_back_out5) -> fir_dbl_col3/26(imag_back5)
  fir_dbl_col4/27(real_back_out6) -> fir_dbl_col3/27(real_back6)
  fir_dbl_col4/28(imag_back_out6) -> fir_dbl_col3/28(imag_back6)
  fir_dbl_col4/29(real_back_out7) -> fir_dbl_col3/29(real_back7)
  fir_dbl_col4/30(imag_back_out7) -> fir_dbl_col3/30(imag_back7)
  fir_dbl_col4/31(real_back_out8) -> fir_dbl_col3/31(real_back8)
  fir_dbl_col4/32(imag_back_out8) -> fir_dbl_col3/32(imag_back8)
  fir_dbl_col5/17(real_back_out1) -> fir_dbl_col4/17(real_back1)
  fir_dbl_col5/18(imag_back_out1) -> fir_dbl_col4/18(imag_back1)
  fir_dbl_col5/19(real_back_out2) -> fir_dbl_col4/19(real_back2)
  fir_dbl_col5/20(imag_back_out2) -> fir_dbl_col4/20(imag_back2)
  fir_dbl_col5/21(real_back_out3) -> fir_dbl_col4/21(real_back3)
  fir_dbl_col5/22(imag_back_out3) -> fir_dbl_col4/22(imag_back3)
  fir_dbl_col5/23(real_back_out4) -> fir_dbl_col4/23(real_back4)
  fir_dbl_col5/24(imag_back_out4) -> fir_dbl_col4/24(imag_back4)
  fir_dbl_col5/25(real_back_out5) -> fir_dbl_col4/25(real_back5)
  fir_dbl_col5/26(imag_back_out5) -> fir_dbl_col4/26(imag_back5)
  fir_dbl_col5/27(real_back_out6) -> fir_dbl_col4/27(real_back6)
  fir_dbl_col5/28(imag_back_out6) -> fir_dbl_col4/28(imag_back6)
  fir_dbl_col5/29(real_back_out7) -> fir_dbl_col4/29(real_back7)
  fir_dbl_col5/30(imag_back_out7) -> fir_dbl_col4/30(imag_back7)
  fir_dbl_col5/31(real_back_out8) -> fir_dbl_col4/31(real_back8)
  fir_dbl_col5/32(imag_back_out8) -> fir_dbl_col4/32(imag_back8)
  fir_dbl_col5/1(real_out1) -> fir_dbl_col5/17(real_back1)
  fir_dbl_col5/2(imag_out1) -> fir_dbl_col5/18(imag_back1)
  fir_dbl_col5/3(real_out2) -> fir_dbl_col5/19(real_back2)
  fir_dbl_col5/4(imag_out2) -> fir_dbl_col5/20(imag_back2)
  fir_dbl_col5/5(real_out3) -> fir_dbl_col5/21(real_back3)
  fir_dbl_col5/6(imag_out3) -> fir_dbl_col5/22(imag_back3)
  fir_dbl_col5/7(real_out4) -> fir_dbl_col5/23(real_back4)
  fir_dbl_col5/8(imag_out4) -> fir_dbl_col5/24(imag_back4)
  fir_dbl_col5/9(real_out5) -> fir_dbl_col5/25(real_back5)
  fir_dbl_col5/10(imag_out5) -> fir_dbl_col5/26(imag_back5)
  fir_dbl_col5/11(real_out6) -> fir_dbl_col5/27(real_back6)
  fir_dbl_col5/12(imag_out6) -> fir_dbl_col5/28(imag_back6)
  fir_dbl_col5/13(real_out7) -> fir_dbl_col5/29(real_back7)
  fir_dbl_col5/14(imag_out7) -> fir_dbl_col5/30(imag_back7)
  fir_dbl_col5/15(real_out8) -> fir_dbl_col5/31(real_back8)
  fir_dbl_col5/16(imag_out8) -> fir_dbl_col5/32(imag_back8)

== system ddc_dev/freq_cwg0 ==
  sim_1 : Inport
  convert1_1 : DataTypeConversion  OutDataTypeStr=fixdt('ufix26_En0')  LockScale=on
  convert2_1 : DataTypeConversion  OutDataTypeStr=fixdt('ufix26_En0')  ConvertRealWorld=Stored Integer (SI)  LockScale=on
  ddc_dev_freq_cwg0_user_data_out : xbsIndex_r4/Gateway In  gui_display_data_type=Fixed-point  arith_type=Unsigned  n_bits=32  bin_pt=0  preci_type=Single  exp_width=8  frac_width=24  rows=1  columns=1  quantization="Round  (unbiased: +/- Inf)"  overflow=Saturate  period=1  UseAsADC=off  ADCChannel='1'  interface=None  automatic_assignment=on  address_offset=hex2dec('00')  intf_name=''  intf_description=''  default_value=0  timing_constraint=None  locs_specified=off  LOCs={}  io_standard={}  inherit_from_input=off  hdl_port=on  dbl_ovrd=off  block_type=gatewayin
  gain_1 : Gain
  io_delay : xbsIndex_r4/Delay  rst=off  infoeditControl=Selection of Reset will increase slice count due to use of real FFs and instead of SRLs  en=off  latency=1  reg_retiming=on  dbl_ovrd=off  block_type=delay
      settings: infoedit=Hardware notes: A delay line is a chain, each link of which is an SRL16 or SRL32 followed by a flip-flop.
  reint1 : xbsIndex_r4/Reinterpret  force_arith_type=on  arith_type=Unsigned  force_bin_pt=on  bin_pt=0  block_type=reinterpret
  slice_frequency : xbsIndex_r4/Slice  nbits=26  boolean_output=off  mode=Lower Bit Location + Width  bit1=0  base1=MSB of Input  bit0=0  base0=LSB of Input  dbl_ovrd=off  block_type=slice
  in_frequency : Outport
  wires:
  ddc_dev_freq_cwg0_user_data_out/1 -> io_delay/1
  sim_1/1 -> convert1_1/1
  convert1_1/1 -> convert2_1/1
  convert2_1/1 -> gain_1/1
  gain_1/1 -> ddc_dev_freq_cwg0_user_data_out/1
  io_delay/1 -> slice_frequency/1
  slice_frequency/1 -> reint1/1
  reint1/1 -> in_frequency/1

== system ddc_dev/freq_cwg_corr ==
  sim_1 : Inport
  convert1_1 : DataTypeConversion  OutDataTypeStr=fixdt('ufix26_En0')  LockScale=on
  convert2_1 : DataTypeConversion  OutDataTypeStr=fixdt('ufix26_En0')  ConvertRealWorld=Stored Integer (SI)  LockScale=on
  ddc_dev_freq_cwg_corr_user_data_out : xbsIndex_r4/Gateway In  gui_display_data_type=Fixed-point  arith_type=Unsigned  n_bits=32  bin_pt=0  preci_type=Single  exp_width=8  frac_width=24  rows=1  columns=1  quantization="Round  (unbiased: +/- Inf)"  overflow=Saturate  period=1  UseAsADC=off  ADCChannel='1'  interface=None  automatic_assignment=on  address_offset=hex2dec('00')  intf_name=''  intf_description=''  default_value=0  timing_constraint=None  locs_specified=off  LOCs={}  io_standard={}  inherit_from_input=off  hdl_port=on  dbl_ovrd=off  block_type=gatewayin
  gain_1 : Gain
  io_delay : xbsIndex_r4/Delay  rst=off  infoeditControl=Selection of Reset will increase slice count due to use of real FFs and instead of SRLs  en=off  latency=1  reg_retiming=on  dbl_ovrd=off  block_type=delay
      settings: infoedit=Hardware notes: A delay line is a chain, each link of which is an SRL16 or SRL32 followed by a flip-flop.
  reint1 : xbsIndex_r4/Reinterpret  force_arith_type=on  arith_type=Unsigned  force_bin_pt=on  bin_pt=0  block_type=reinterpret
  slice_frequency : xbsIndex_r4/Slice  nbits=26  boolean_output=off  mode=Lower Bit Location + Width  bit1=0  base1=MSB of Input  bit0=0  base0=LSB of Input  dbl_ovrd=off  block_type=slice
  in_frequency : Outport
  wires:
  ddc_dev_freq_cwg_corr_user_data_out/1 -> io_delay/1
  sim_1/1 -> convert1_1/1
  convert1_1/1 -> convert2_1/1
  convert2_1/1 -> gain_1/1
  gain_1/1 -> ddc_dev_freq_cwg_corr_user_data_out/1
  io_delay/1 -> slice_frequency/1
  slice_frequency/1 -> reint1/1
  reint1/1 -> in_frequency/1

== system ddc_dev/mixer ==
  sync : Inport
  din1 : Inport  Port=2
  dds : Subsystem  AncestorBlock=casper_library_downconverter/dds  mask(dds){freq_div=16, freq=1, num_lo=1, n_bits=10, latency=2}
      mask prompts: freq_div "Frequency divisions (M)"; freq "Frequency (? / M*2pi)"; num_lo "Parallel LOs"; n_bits "Bit Width"
      mask help:
      | Generates P channels of sin and cos data for mixing
      | with input data in a DDC. To generate frequency
      | N/M(Fc x P) (where Fc is the clock rate)
      | M = "Frequency Divisions", N = "Frequency",
      | Parallel LOs = P
      mask init:
      | dds_init(gcb, ...
      |     'freq_div', freq_div, ...
      |     'freq', freq, ...
      |     'num_lo', num_lo, ...
      |     'n_bits', n_bits, ...
      |     'latency', latency);
      settings: AttributesFormatString=lo at -1/16
      mask Help: eval('xlWeb(''http://casper.berkeley.edu/wiki/Dds'')')
  delay : xbsIndex_r4/Delay  rst=off  infoeditControl=Selection of Reset will increase slice count due to use of real FFs and instead of SRLs  en=off  latency=4  reg_retiming=off  dbl_ovrd=off  block_type=delay
      settings: infoedit=Hardware notes: A delay line is a chain, each link of which is an SRL16 or SRL32 followed by a flip-flop.
  rcmult1 : Subsystem  AncestorBlock=casper_library_downconverter/rcmult  mask(rcmult){latency=4}
      mask prompts: latency "Multiplier latency"
      mask help:
      | Multiplies input data with cos and sin inputs and
      | outputs results on real and imag ports
      | respectively.
      mask init:
      | rcmult_init(gcb, ...
      |     'latency', latency);
      mask Help: eval('xlWeb(''http://casper.berkeley.edu/wiki/Rcmult'')')
  sync_out : Outport
  real1 : Outport  Port=2
  imag1 : Outport  Port=3
  wires:
  sync/1 -> delay/1, dds/1(sync)
  delay/1 -> sync_out/1
  din1/1 -> rcmult1/1(d)
  dds/1(sin0) -> rcmult1/2(sin)
  dds/2(cos0) -> rcmult1/3(cos)
  rcmult1/1(real) -> real1/1
  rcmult1/2(imag) -> imag1/1

== system ddc_dev/pipeline147 ==
  d : Inport
  Register0 : xbsIndex_r4/Register  init=0  rst=off  en=off  dbl_ovrd=off  block_type=register
      settings: block_version=11.4
  Register1 : xbsIndex_r4/Register  init=0  rst=off  en=off  dbl_ovrd=off  block_type=register
      settings: block_version=11.4
  q : Outport
  wires:
  Register1/1 -> q/1
  d/1 -> Register0/1
  Register0/1 -> Register1/1

== system ddc_dev/pipeline156 ==
  d : Inport
  Register0 : xbsIndex_r4/Register  init=0  rst=off  en=off  dbl_ovrd=off  block_type=register
      settings: block_version=11.4
  Register1 : xbsIndex_r4/Register  init=0  rst=off  en=off  dbl_ovrd=off  block_type=register
      settings: block_version=11.4
  q : Outport
  wires:
  Register1/1 -> q/1
  d/1 -> Register0/1
  Register0/1 -> Register1/1

== system ddc_dev/pipeline161 ==
  d : Inport
  Register0 : xbsIndex_r4/Register  init=0  rst=off  en=off  dbl_ovrd=off  block_type=register
      settings: block_version=11.4
  Register1 : xbsIndex_r4/Register  init=0  rst=off  en=off  dbl_ovrd=off  block_type=register
      settings: block_version=11.4
  q : Outport
  wires:
  Register1/1 -> q/1
  d/1 -> Register0/1
  Register0/1 -> Register1/1

== system ddc_dev/pipeline162 ==
  d : Inport
  Register0 : xbsIndex_r4/Register  init=0  rst=off  en=off  dbl_ovrd=off  block_type=register
      settings: block_version=11.4
  Register1 : xbsIndex_r4/Register  init=0  rst=off  en=off  dbl_ovrd=off  block_type=register
      settings: block_version=11.4
  q : Outport
  wires:
  Register1/1 -> q/1
  d/1 -> Register0/1
  Register0/1 -> Register1/1
